simulink model "Modular_Model_New_Board"  (R2018a)
settings: Solver=FixedStepAuto  StartTime=0.0  StopTime=Tfinal  FixedStep=SampleTime*1e-2  MinStep=SampleTime*1e-2  RelTol=1e-3
values from neighbouring files (symbols this model uses):
  ESRA = 21.1e-3    (= 0.0211)    [sim_param_new_board.m]
  ESRB = 21.1e-3    (= 0.0211)    [sim_param_new_board.m]
  ESRC = 21.1e-3    (= 0.0211)    [sim_param_new_board.m]
  ffund = 50    [sim_param_new_board.m]
  LAMid = 01.30e-9    (= 1.3e-09)    [sim_param_new_board.m]
  LBMid = 01.30e-9    (= 1.3e-09)    [sim_param_new_board.m]
  LCMid = 01.30e-9    (= 1.3e-09)    [sim_param_new_board.m]
  ModulationIndex1 = 0.9    [sim_param_new_board.m]
  Module1Phase = 0    [sim_param_new_board.m]
  RABBot = 10.20e-9    (= 1.02e-08)    [sim_param_new_board.m]
  RABot = 20.25e-9    (= 2.025e-08)    [sim_param_new_board.m]
  RABTop = 18.30e-9    (= 1.83e-08)    [sim_param_new_board.m]
  RAMid = 01.30e-9    (= 1.3e-09)    [sim_param_new_board.m]
  RATop = 03.40e-9    (= 3.4e-09)    [sim_param_new_board.m]
  RBBot = 20.38e-9    (= 2.038e-08)    [sim_param_new_board.m]
  RBCBot = 11.14e-9    (= 1.114e-08)    [sim_param_new_board.m]
  RBCTop = 21.84e-9    (= 2.184e-08)    [sim_param_new_board.m]
  RBMid = 01.30e-9    (= 1.3e-09)    [sim_param_new_board.m]
  RBTop = 03.38e-9    (= 3.38e-09)    [sim_param_new_board.m]
  RCBot = 20.94e-9    (= 2.094e-08)    [sim_param_new_board.m]
  RCMid = 01.30e-9    (= 1.3e-09)    [sim_param_new_board.m]
  RCTop = 03.41e-9    (= 3.41e-09)    [sim_param_new_board.m]
  Rin = 0.1    [sim_param_new_board.m]
  Rload1 = Z1*PF    [sim_param_new_board.m]
  Vmodule = 270    [sim_param_new_board.m]
  VpulseMax = 6    [sim_param_new_board.m]
  VpulseMin = -3    [sim_param_new_board.m]
libraries: elec_lib x81, fl_lib x38, nesl_utility x38, simulink x12, powerlib_meascontrol x4
(part 1 of 3)
settings Model: SimulationMode=accelerator  Creator=Furkan  LastModifiedBy=enes_
settings DataIOCC: SaveOutput=off  SignalLogging=off  DSMLogging=off  SaveTime=off
settings OptimizationCC: LifeSpan=inf
settings DebuggingCC: SFExecutionAtInitializationDiag=none
settings CodeAppCC: StateflowObjectComments=on
settings SimscapeCC: SimscapeNormalizeSystem=off

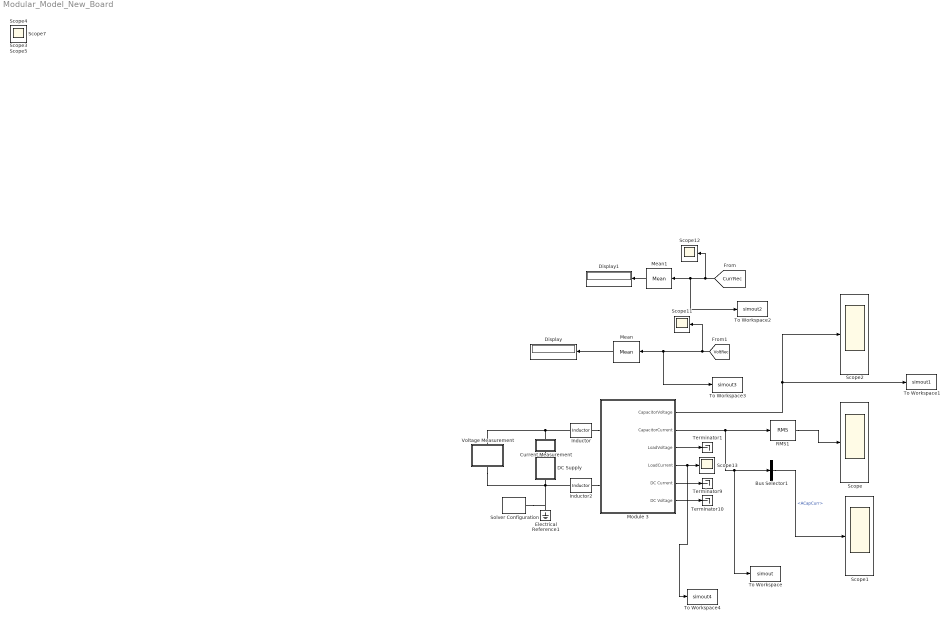
== system Modular_Model_New_Board ==
  Bus Selector1 : BusSelector  OutputSignals=ACapCurr
  "Current Measurement " : Subsystem
  DC Supply : Subsystem
  Display : Display
  Display1 : Display
  Electrical Reference1 : fl_lib/Electrical/Electrical Elements/Electrical Reference
  Inductor : elec_lib/Passive Devices/Inductor  l=POS1 H  L_tol=20  enable_L_tol=0  tol_distribution=1  nSigma=4  r=0 Ohm  g=1e-9 1/Ohm  enable_operating_limits=0  operating_limit_action=2  max_working_current=1 A  power_rating=1 W  enable_faults=0  fault_action=1  lambdaPercent=50  k_faulted=0.9999  turnsShort=0  openCct=0  groundShort=0  groundShortG=0 1/Ohm  tau_fault=1e-3 s  enable_temporal_fault=0  t_fault=1 s  enable_behavioral_fault=0  max_permissible_voltage=100 V  n_fail_on_voltage=1  max_permissible_current=1 A  t_fail_on_current=1 s  i_L_specify=on  i_L_priority=High  i_L=0 A  i_L_nominal_specify=off  i_L_nominal_unit=A  i_L_nominal_value=1
      settings: SourceProductName=Simscape Electronics  SourceProductBaseCode=SN
  Inductor2 : elec_lib/Passive Devices/Inductor  l=NEG1 H  L_tol=20  enable_L_tol=0  tol_distribution=1  nSigma=4  r=0 Ohm  g=1e-9 1/Ohm  enable_operating_limits=0  operating_limit_action=2  max_working_current=1 A  power_rating=1 W  enable_faults=0  fault_action=1  lambdaPercent=50  k_faulted=0.9999  turnsShort=0  openCct=0  groundShort=0  groundShortG=0 1/Ohm  tau_fault=1e-3 s  enable_temporal_fault=0  t_fault=1 s  enable_behavioral_fault=0  max_permissible_voltage=100 V  n_fail_on_voltage=1  max_permissible_current=1 A  t_fail_on_current=1 s  i_L_specify=on  i_L_priority=High  i_L=0 A  i_L_nominal_specify=off  i_L_nominal_unit=A  i_L_nominal_value=1
      settings: SourceProductName=Simscape Electronics  SourceProductBaseCode=SN
  Mean : powerlib_meascontrol/Measurements/Mean  Freq=ffund  Vinit=0  Ts=0
  Mean1 : powerlib_meascontrol/Measurements/Mean  Freq=ffund  Vinit=0  Ts=0
  Module 3 : Subsystem
  RMS1 : powerlib_meascontrol/Measurements/RMS  TrueRMS=on  Freq=40000  RMSInit=0  Ts=0
  Scope{,1..5,7,11..13} (10 alike) : Scope
  Solver Configuration : nesl_utility/Solver Configuration  PhysicalDomain=network_engine_domain  SubClassName=solver  LeftPortType=input  RightPortType=generic  Tones=[]  Harmonics=[]  SimulateNoise=off  Profile=off  UseLocalSampling=off  EnableSwitchedLinearOptims=on  FrequencyDomain=off  UseCCode=off  RelTol=0.001  AbsTol=1e-06  MinStep=1e-09  ToWorkspace=off  RevertToSquareIcSolve=off  NumHomotopyIterations=100  PhasorMode=off  PhasorModeNumHarmonics=1  DoDC=off  ResidualTolerance=1e-09  UseLocalSolver=on  LocalSolverChoice=NE_BACKWARD_EULER_ADVANCER  LocalSolverSampleTime=SampleTime  DoFixedCost=on  MaxNonlinIter=3  MaxModeIter=2  LinearAlgebra=Sparse  EquationFormulation=NE_TIME_EF  DelaysMemoryBudget=1024  AutomaticFiltering=on  FilteringTimeConstant=0.001
  Terminator1 : Terminator
  Terminator10 : Terminator
  Terminator9 : Terminator
  To Workspace : ToWorkspace  VariableName=simout  SaveFormat=Timeseries  SampleTime=-1
  To Workspace1 : ToWorkspace  VariableName=simout1  SaveFormat=Timeseries  SampleTime=-1
  To Workspace2 : ToWorkspace  VariableName=simout2  SaveFormat=Timeseries  SampleTime=-1
  To Workspace3 : ToWorkspace  VariableName=simout3  SaveFormat=Timeseries  SampleTime=-1
  To Workspace4 : ToWorkspace  VariableName=simout4  SaveFormat=Timeseries  SampleTime=-1
  Voltage Measurement : Subsystem
  wires:
  Module 3/1(CapacitorVoltage) -> To Workspace1/1, Scope2/1
  Module 3/2(CapacitorCurrent) -> To Workspace/1, Bus Selector1/1, RMS1/1
  Module 3/5(DC Current) -> Terminator9/1
  Module 3/6(DC Voltage) -> Terminator10/1
  Bus Selector1/1 -> Scope1/1  "<ACapCurr>"
  Mean/1 -> Display/1
  Mean1/1 -> Display1/1
  Module 3/3(LoadVoltage) -> Terminator1/1
  Module 3/4(LoadCurrent) -> To Workspace4/1, Scope13/1
  [CurrRec] -> Scope12/1, To Workspace2/1, Mean1/1
  [VoltRec] -> Scope11/1, To Workspace3/1, Mean/1
  RMS1/1 -> Scope/1
  connections:
  Inductor2/RConn1 -- Module 3/LConn2
  Inductor/RConn1 -- Module 3/LConn1
  Inductor2/LConn1 -- Electrical Reference1/LConn1 -- Solver Configuration/RConn1 -- Voltage Measurement/RConn1 -- DC Supply/LConn1
  "Current Measurement "/RConn1 -- Voltage Measurement/LConn1 -- Inductor/LConn1
  "Current Measurement "/LConn1 -- DC Supply/RConn1

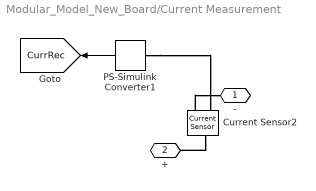
== system Modular_Model_New_Board/Current Measurement  ==
  Current Sensor2 : fl_lib/Electrical/Electrical Sensors/Current Sensor
  PS-Simulink Converter1 : nesl_utility/PS-Simulink Converter  PhysicalDomain=network_engine_domain  SubClassName=ps_output  LeftPortType=input  RightPortType=output  PseudoPeriodic=off  Frequencies=[]  Unit=1  AffineConversion=off
  - : PMIOPort  Side=Right
  + : PMIOPort  Port=2  Side=Left
  tag scope: CurrRec=global
  wires:
  PS-Simulink Converter1/1 -> [CurrRec]
  connections:
  PS-Simulink Converter1/LConn1 -- Current Sensor2/RConn1
  Current Sensor2/LConn1 -- +/RConn1
  Current Sensor2/RConn2 -- -/RConn1

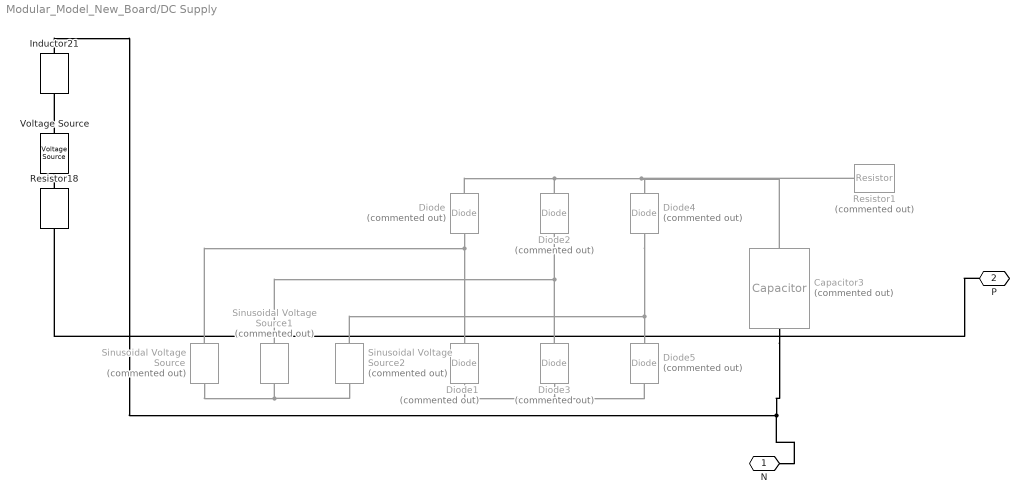
== system Modular_Model_New_Board/DC Supply ==
  Capacitor3 : elec_lib/Passive Devices/Capacitor  Commented=on  enable_table=0  c=5 mF  Cvec=[1e-05, 1e-06] F  Vvec=[0, 10] V  CV_table_symmetry=1  C_tol=0  enable_C_tol=0  tol_distribution=1  nSigma=4  r=21.1e-3 Ohm  g=0 1/Ohm  enable_operating_limits=0  operating_limit_action=2  max_working_voltage_range=[-25, 25] V  power_rating=1 W  enable_faults=0  fault_action=1  Cscale_faulted=100  R_faulted=1e-3 Ohm  G_faulted=0 1/Ohm  tau_fault=1e-3 s  enable_temporal_fault=0  t_fault=1 s  enable_behavioral_fault=0  max_permissible_voltage_range=[-100, 100] V  t_fail_on_voltage=1 s  i_specify=off  i_priority=None  i=0 A  i_nominal_specify=off  i_nominal_unit=A  i_nominal_value=1  v_specify=off  v_priority=None  v=0 V  v_nominal_specify=off  v_nominal_unit=V  v_nominal_value=1  vc_specify=on  vc_priority=High  vc=270 V  vc_nominal_specify=off  vc_nominal_unit=V  vc_nominal_value=1
  Diode{,1..5} (6 alike) : elec_lib/Semiconductor Devices/Diode  Commented=on  ModelType=1  Vf=0.6 V  Ron=0.3 Ohm  Goff=1e-8 S  Rz=0.3 Ohm  Vz=50 V  C_PWL=5 pF  prmExp=1  I12=[.0137, .545] A  V12=[.6, .7] V  I1=0.0137 A  V1=0.6 V  IS=1e-12 A  ec=1  RS=0.01 Ohm  Tmeas=25 degC  BV=inf V  C_param=1  CJ0=5 pF  VJ=1 V  Mgrad=0.5  Vvec=[.1, 10, 100] V  Cvec=[3.5, 1, .4] pF  FC=0.5  Q_param=1  Irrm=-7.15 A  iF=4 A  didt=-750 A/us  trr=115 ns  TT=50 ns  tau=100 ns  T_param=1  IS_T2=1.25e-7 A  I1_T2=0.245 A  V1_T2=0.5 V  Tmeas2=125 degC  EG_param=1  EG=1.11 eV  XTI_param=1  XTI=3  dBVdT=0 V/K  Tdevice=25 degC  i_capacitor_specify=off  i_capacitor_priority=High  i_capacitor=0 A  i_capacitor_nominal_specify=off  i_capacitor_nominal_unit=A  i_capacitor_nominal_value=1  v_capacitor_specify=off  v_capacitor_priority=None  v_capacitor=0 V  v_capacitor_nominal_specify=off  v_capacitor_nominal_unit=V  v_capacitor_nominal_value=1  Rth=[0, 10] K/W  thermal_mass_parameterization=1  thermal_mass=[0, 1] J/K  thermal_time_constant=[0, 10] s  thermal_mass_initial_temperatures=[25, 25] degC
      settings: SourceProductName=Simscape Electronics  SourceProductBaseCode=SN
  Inductor21 : elec_lib/Passive Devices/Inductor  l=Lin H  L_tol=20  enable_L_tol=0  tol_distribution=1  nSigma=4  r=0 Ohm  g=1e-9 1/Ohm  enable_operating_limits=0  operating_limit_action=2  max_working_current=1 A  power_rating=1 W  enable_faults=0  fault_action=1  lambdaPercent=50  k_faulted=0.9999  turnsShort=0  openCct=0  groundShort=0  groundShortG=0 1/Ohm  tau_fault=1e-3 s  enable_temporal_fault=0  t_fault=1 s  enable_behavioral_fault=0  max_permissible_voltage=100 V  n_fail_on_voltage=1  max_permissible_current=1 A  t_fail_on_current=1 s  i_L_specify=on  i_L_priority=High  i_L=0 A  i_L_nominal_specify=off  i_L_nominal_unit=A  i_L_nominal_value=1
      settings: SourceProductName=Simscape Electronics  SourceProductBaseCode=SN
  Resistor1 : elec_lib/Passive Devices/Resistor  Commented=on  R=Rin Ohm  R_tol=1  enable_R_tol=0  tol_distribution=1  nSigma=4  enable_operating_limits=0  operating_limit_action=2  max_working_voltage=100 V  power_rating=1 W  enable_faults=0  fault_action=1  R_faulted=inf Ohm  enable_temporal_fault=0  t_fault=1 s  enable_behavioral_fault=0  max_permissible_current=1 A  t_fail_on_current=1 s  noise_mode=0  sample_time=1e-3 s  repeatability=1  auto_seed=1378460567  user_seed=0  Tdevice=25 degC  alpha=3.93e-3 1/K  Tmeas=25 degC  thermal_mass=100 J/K  power_derating_T1=70 degC  power_derating_T2=155 degC  operating_temperature_range_vec=[-50, 150] degC  temperature_specify=off  temperature_priority=High  temperature=298.15 K  temperature_nominal_specify=off  temperature_nominal_unit=K  temperature_nominal_value=1
  Resistor18 : elec_lib/Passive Devices/Resistor  R=Rin Ohm  R_tol=1  enable_R_tol=0  tol_distribution=1  nSigma=4  enable_operating_limits=0  operating_limit_action=2  max_working_voltage=100 V  power_rating=1 W  enable_faults=0  fault_action=1  R_faulted=inf Ohm  enable_temporal_fault=0  t_fault=1 s  enable_behavioral_fault=0  max_permissible_current=1 A  t_fail_on_current=1 s  noise_mode=0  sample_time=1e-3 s  repeatability=1  auto_seed=2283412897  user_seed=0  Tdevice=25 degC  alpha=3.93e-3 1/K  Tmeas=25 degC  thermal_mass=100 J/K  power_derating_T1=70 degC  power_derating_T2=155 degC  operating_temperature_range_vec=[-50, 150] degC  temperature_specify=off  temperature_priority=High  temperature=298.15 K  temperature_nominal_specify=off  temperature_nominal_unit=K  temperature_nominal_value=1
  Sinusoidal Voltage Source : elec_lib/Additional Components/SPICE-Compatible Components/Sources/Sinusoidal Voltage Source  Commented=on  VO=0 V  VA=Vin V  FREQ=50 Hz  TD=0 s  DF=0 1/s  OMEGA=0 rad/s
      settings: SourceProductName=Simscape Electronics  SourceProductBaseCode=SN
  Sinusoidal Voltage Source1 : elec_lib/Additional Components/SPICE-Compatible Components/Sources/Sinusoidal Voltage Source  Commented=on  VO=0 V  VA=Vin V  FREQ=50 Hz  TD=2/150 s  DF=0 1/s  OMEGA=0 rad/s
      settings: SourceProductName=Simscape Electronics  SourceProductBaseCode=SN
  Sinusoidal Voltage Source2 : elec_lib/Additional Components/SPICE-Compatible Components/Sources/Sinusoidal Voltage Source  Commented=on  VO=0 V  VA=Vin V  FREQ=50 Hz  TD=1/150 s  DF=0 1/s  OMEGA=0 rad/s
      settings: SourceProductName=Simscape Electronics  SourceProductBaseCode=SN
  Voltage Source : elec_lib/Sources/Voltage Source  dc_voltage=Vin V  ac_voltage=0 V  ac_shift=0 rad  ac_frequency=60 Hz  noise_mode=0  PSD=0 V^2/Hz  repeatability=1  auto_seed=3750339491  user_seed=0  sample_time=1e-3 s  i_specify=off  i_priority=None  i=0 A  i_nominal_specify=off  i_nominal_unit=A  i_nominal_value=1  v_specify=off  v_priority=None  v=0 V  v_nominal_specify=off  v_nominal_unit=V  v_nominal_value=1
      settings: SourceProductName=Simscape Electronics  SourceProductBaseCode=SN
  N : PMIOPort  Side=Left
  P : PMIOPort  Port=2  Side=Right
  connections:
  P/RConn1 -- Resistor18/RConn1
  Sinusoidal Voltage Source/RConn1 -- Sinusoidal Voltage Source2/RConn1 -- Sinusoidal Voltage Source1/RConn1
  Diode/RConn1 -- Diode2/RConn1 -- Resistor1/LConn1 -- Capacitor3/LConn1 -- Diode4/RConn1
  Diode/LConn1 -- Sinusoidal Voltage Source/LConn1 -- Diode1/RConn1
  Diode3/RConn1 -- Sinusoidal Voltage Source1/LConn1 -- Diode2/LConn1
  Diode4/LConn1 -- Sinusoidal Voltage Source2/LConn1 -- Diode5/RConn1
  N/RConn1 -- Capacitor3/RConn1 -- Inductor21/LConn1
  Resistor18/LConn1 -- Voltage Source/LConn1
  Voltage Source/RConn1 -- Inductor21/RConn1
  Diode1/LConn1 -- Diode3/LConn1 -- Diode5/LConn1
